simulink model "HW3_P4"  (R2017a)
settings: Solver=VariableStepAuto  StartTime=0.0  StopTime=10.0  RelTol=1e-3
settings Model: Creator=Merc  LastModifiedBy=Merc

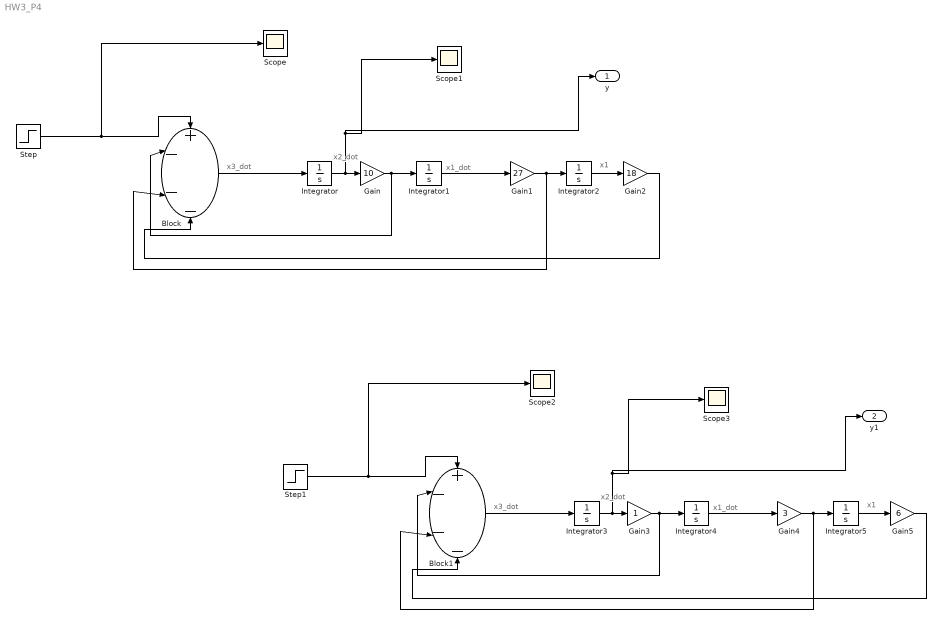
== system HW3_P4 ==
  note: x1
  note: x1_dot
  note: x2_dot
  note: x3_dot
  note: x1
  note: x2_dot
  note: x3_dot
  note: x1_dot
  Block : Sum  Inputs=+---
  Block1 : Sum  Inputs=+---
  Gain : Gain  Gain=10
  Gain1 : Gain  Gain=27
  Gain2 : Gain  Gain=18
  Gain3 : Gain
  Gain4 : Gain  Gain=3
  Gain5 : Gain  Gain=6
  Integrator{,1..5} (6 alike) : Integrator
  Scope{,1..3} (4 alike) : Scope
  Step : Step  SampleTime=5
  Step1 : Step  SampleTime=5
  y : Outport  SignalName=y
  y1 : Outport  Port=2  SignalName=y
  wires:
  Block/1 -> Integrator/1
  Integrator/1 -> Scope1/1, y/1, Gain/1
  Gain/1 -> Integrator1/1, Block/2
  Integrator1/1 -> Gain1/1
  Gain1/1 -> Block/3, Integrator2/1
  Integrator2/1 -> Gain2/1
  Gain2/1 -> Block/4
  Step/1 -> Block/1, Scope/1
  Integrator4/1 -> Gain4/1
  Gain5/1 -> Block1/4
  Step1/1 -> Block1/1, Scope2/1
  Integrator5/1 -> Gain5/1
  Block1/1 -> Integrator3/1
  Gain4/1 -> Block1/3, Integrator5/1
  Gain3/1 -> Integrator4/1, Block1/2
  Integrator3/1 -> Scope3/1, y1/1, Gain3/1
